simulink model "GenChassis02"  (Simulink 8.3)
settings: Solver=ode45  StartTime=0.0  StopTime=10.0  RelTol=1e-3
model workspace (MAT data in the model file):
  Chassis.vMass = 1000
  Chassis.vCd = 0.25
  Chassis.frontalArea = 1
  Chassis.airRho = 1.2
  Chassis.tRadius = 0.3
  Chassis.initSpeed = 10
  Chassis.initPosn = 0
  Chassis.brkFactor : numeric (value not decoded)
settings Model: Creator=swami  LastModifiedBy=swami
settings DataIOCC: SignalLoggingSaveFormat=Dataset
settings DebuggingCC: UnderspecifiedInitializationDetection=Simplified  StateNameClashWarn=none
settings GRTTargetCC: CombineOutputUpdateFcns=on  GRTInterface=off

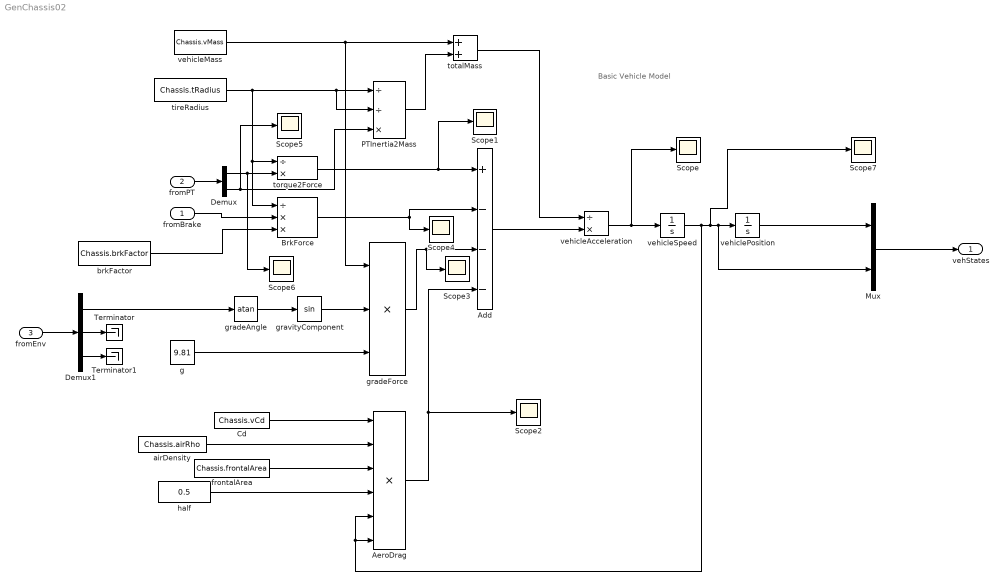
== system GenChassis02 ==
  note: Basic Vehicle Model
  fromBrake : Inport
  fromPT : Inport  Port=2  PortDimensions=2
  fromEnv : Inport  Port=3
  Add : Sum  Inputs=+---
  AeroDrag : Product  Inputs=******
  BrkForce : Product  Inputs=/**
  Cd : Constant  Value=Chassis.vCd
  Demux : Demux  Outputs=2
  Demux1 : Demux  Outputs=3
  Mux : Mux  Inputs=2
  PTInertia2Mass : Product  Inputs=//*
  Scope{,1..7} (8 alike) : Scope
      Scope2 settings: SaveName=ScopeData2
      Scope3 settings: SaveName=ScopeData3
      Scope4 settings: SaveName=ScopeData4
      Scope5 settings: SaveName=ScopeData5
      Scope6 settings: SaveName=ScopeData6
      Scope7 settings: SaveName=ScopeData7
  Terminator : Terminator
  Terminator1 : Terminator
  airDensity : Constant  Value=Chassis.airRho
  brkFactor : Constant  Value=Chassis.brkFactor
  frontalArea : Constant  Value=Chassis.frontalArea
  g : Constant  Value=9.81
  gradeAngle : Trigonometry  Operator=atan
  gradeForce : Product  Inputs=***
  gravityComponent : Trigonometry
  half : Constant  Value=0.5
  tireRadius : Constant  Value=Chassis.tRadius
  torque2Force : Product  Inputs=/*
  totalMass : Sum
  vehicleAcceleration : Product  Inputs=/*
  vehicleMass : Constant  Value=Chassis.vMass
  vehiclePosition : Integrator  InitialCondition=Chassis.initPosn
  vehicleSpeed : Integrator  InitialCondition=Chassis.initSpeed
  vehStates : Outport
  wires:
  fromPT/1 -> Demux/1
  vehicleAcceleration/1 -> Scope/1, vehicleSpeed/1
  vehicleSpeed/1 -> AeroDrag/5, AeroDrag/6, Scope7/1, Mux/2, vehiclePosition/1
  Cd/1 -> AeroDrag/1
  AeroDrag/1 -> Scope2/1, Add/4
  gradeAngle/1 -> gravityComponent/1
  vehicleMass/1 -> gradeForce/1, totalMass/1
  gradeForce/1 -> Scope3/1, Add/3
  gravityComponent/1 -> gradeForce/2
  g/1 -> gradeForce/3
  tireRadius/1 -> BrkForce/1, torque2Force/1, PTInertia2Mass/2, PTInertia2Mass/1
  Demux/2 -> Scope5/1, PTInertia2Mass/3
  Demux/1 -> Scope6/1, torque2Force/2
  torque2Force/1 -> Scope1/1, Add/1
  PTInertia2Mass/1 -> totalMass/2
  totalMass/1 -> vehicleAcceleration/1
  Add/1 -> vehicleAcceleration/2
  BrkForce/1 -> Add/2, Scope4/1
  fromBrake/1 -> BrkForce/2
  airDensity/1 -> AeroDrag/2
  frontalArea/1 -> AeroDrag/3
  half/1 -> AeroDrag/4
  vehiclePosition/1 -> Mux/1
  Mux/1 -> vehStates/1
  fromEnv/1 -> Demux1/1
  Demux1/1 -> gradeAngle/1
  Demux1/2 -> Terminator/1
  Demux1/3 -> Terminator1/1
  brkFactor/1 -> BrkForce/3
